simulink model "archiving_task"  (Simulink 3.00)
libraries: mathlib x4, arclib x3, genlib x2

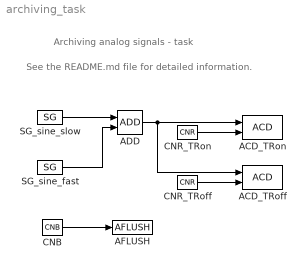
== system archiving_task ==
  note: See the README.md file for detailed information.
  note: Archiving analog signals - task
  ACD_TRoff : arclib/ACD  acls=8: Double  arc=1  id=2  tmin=0.1  tmax=5  TR=off  Desc=Simulated analog signal, TR=off
  ACD_TRon : arclib/ACD  acls=8: Double  arc=1  id=1  tmin=0.1  tmax=5  TR=on  Desc=Simulated analog signal, TR=on
  ADD : mathlib/ADD
  AFLUSH : arclib/AFLUSH  arc=1
  CNB : mathlib/CNB  YCN=off
  CNR_TRoff : mathlib/CNR  ycn=0.2
  CNR_TRon : mathlib/CNR  ycn=0.2
  SG_sine_fast : genlib/SG  isig=1: SINE  amp=3  freq=0.09  phase=0  ifrunit=1: Hz  iphunit=1: degrees  offset=0
  SG_sine_slow : genlib/SG  isig=1: SINE  amp=10  freq=0.025  phase=0  ifrunit=1: Hz  iphunit=1: degrees  offset=0
  wires:
  ADD/1 -> ACD_TRoff/1, ACD_TRon/1
  CNB/1 -> AFLUSH/1
  CNR_TRoff/1 -> ACD_TRoff/2
  CNR_TRon/1 -> ACD_TRon/2
  SG_sine_fast/1 -> ADD/2
  SG_sine_slow/1 -> ADD/1
